simulink model "bid"  (R2015b)
settings: Solver=ode45  SolverMode=SingleTasking  StartTime=0.0  StopTime=10.0  RelTol=1e-3
undefined symbols (not defined in the file or in its folder): l1, rho1
libraries: cstblocks x1
settings Model: Creator=d.alazard  LastModifiedBy=d.alazard
settings DataIOCC: SaveFormat=Array
settings OptimizationCC: BlockReduction=off  BooleanDataType=off
settings DebuggingCC: SaveWithParameterizedLinksMsg=none  UnderspecifiedInitializationDetection=Classic  MergeDetectMultiDrivingBlocksExec=none  SignalResolutionControl=TryResolveAllWithWarning
settings HardwareCC: ProdBitPerPointer=32  ProdLargestAtomicFloat=None  ProdIntDivRoundTo=Undefined  ProdEndianess=Unspecified  ProdWordSize=32  ProdHWDeviceType=32-bit Generic  TargetUnknown=on
settings GRTTargetCC: GeneratePreprocessorConditionals=Disable all
settings ConfigComp: CovModelRefEnable=Off  CovSFcnEnable=off

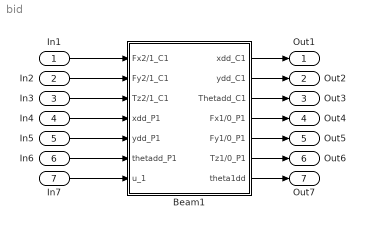
== system bid ==
  In1 : Inport
  In2 : Inport  Port=2
  In3 : Inport  Port=3
  In4 : Inport  Port=4
  In5 : Inport  Port=5
  In6 : Inport  Port=6
  In7 : Inport  Port=7
  Beam1 : Subsystem
  Out1 : Outport
  Out2 : Outport  Port=2
  Out3 : Outport  Port=3
  Out4 : Outport  Port=4
  Out5 : Outport  Port=5
  Out6 : Outport  Port=6
  Out7 : Outport  Port=7
  wires:
  In6/1 -> Beam1/6(thetadd_P1)
  In5/1 -> Beam1/5(ydd_P1)
  In4/1 -> Beam1/4(xdd_P1)
  In3/1 -> Beam1/3(Tz2/1_C1)
  In2/1 -> Beam1/2(Fy2/1_C1)
  In1/1 -> Beam1/1(Fx2/1_C1)
  In7/1 -> Beam1/7(u_1)
  Beam1/6(Tz1/0_P1) -> Out6/1
  Beam1/7(theta1dd) -> Out7/1
  Beam1/5(Fy1/0_P1) -> Out5/1
  Beam1/4(Fx1/0_P1) -> Out4/1
  Beam1/3(Thetadd_C1) -> Out3/1
  Beam1/1(xdd_C1) -> Out1/1
  Beam1/2(ydd_C1) -> Out2/1

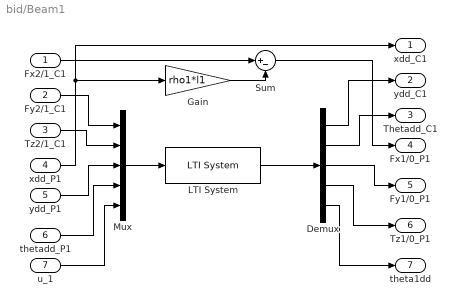
== system bid/Beam1 ==
  Fx2/1_C1 : Inport
  Fy2/1_C1 : Inport  Port=2
  Tz2/1_C1 : Inport  Port=3
  xdd_P1 : Inport  Port=4
  ydd_P1 : Inport  Port=5
  thetadd_P1 : Inport  Port=6
  u_1 : Inport  Port=7
  Demux : Demux  Outputs=5
  Gain : Gain  Gain=rho1*l1
  LTI System : cstblocks/LTI System  sys=Mam1_5  IC=[]
  Mux : Mux  Inputs=5
  Sum : Sum  Inputs=|+-
  xdd_C1 : Outport
  ydd_C1 : Outport  Port=2
  Thetadd_C1 : Outport  Port=3
  Fx1/0_P1 : Outport  Port=4
  Fy1/0_P1 : Outport  Port=5
  Tz1/0_P1 : Outport  Port=6
  theta1dd : Outport  Port=7
  wires:
  u_1/1 -> Mux/5
  Demux/5 -> theta1dd/1
  LTI System/1 -> Demux/1
  Demux/4 -> Tz1/0_P1/1
  ydd_P1/1 -> Mux/3
  Fy2/1_C1/1 -> Mux/1
  Tz2/1_C1/1 -> Mux/2
  thetadd_P1/1 -> Mux/4
  Demux/1 -> ydd_C1/1
  Demux/2 -> Thetadd_C1/1
  Demux/3 -> Fy1/0_P1/1
  Mux/1 -> LTI System/1
  xdd_P1/1 -> Gain/1, xdd_C1/1
  Fx2/1_C1/1 -> Sum/1
  Sum/1 -> Fx1/0_P1/1
  Gain/1 -> Sum/2
